simulink model "main"  (Simulink 7.3)
settings: Solver=ode45  StartTime=0.0  StopTime=10.0  RelTol=1e-7
libraries: simulink x2
settings Model: Creator=Sain  LastModifiedBy=Sain

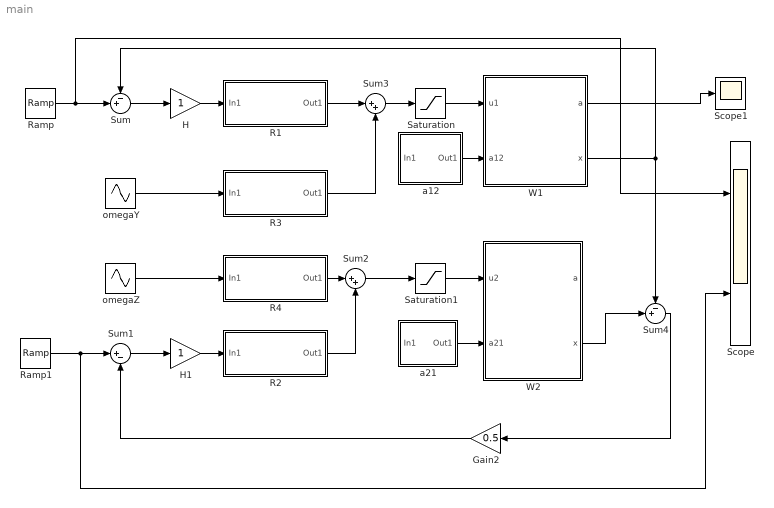
== system main ==
  Gain2 : Gain  Gain=0.5  ParameterDataType=fixdt(1, 16)  ParameterScaling=2^0  OutDataType=fixdt(1, 16)  OutScaling=2^0
  H : Gain  ParameterDataType=fixdt(1, 16)  ParameterScaling=2^0  OutDataType=fixdt(1, 16)  OutScaling=2^0
  H1 : Gain  ParameterDataType=fixdt(1, 16)  ParameterScaling=2^0  OutDataType=fixdt(1, 16)  OutScaling=2^0
  R1 : Subsystem
  R2 : Subsystem
  R3 : Subsystem
  R4 : Subsystem
  Ramp : simulink/Sources/Ramp  SystemSampleTime=-1  slope=60  start=1  X0=0
  Ramp1 : simulink/Sources/Ramp  SystemSampleTime=-1  slope=30  start=2  X0=0
  Saturation : Saturate  UpperLimit=27  LowerLimit=-27  OutDataType=fixdt(1, 16)  OutScaling=2^0
  Saturation1 : Saturate  UpperLimit=27  LowerLimit=-27  OutDataType=fixdt(1, 16)  OutScaling=2^0
  Scope : Scope  NumInputPorts=2
      settings: YMin=-5~-5  YMax=5~5
  Scope1 : Scope
  Sum : Sum  Inputs=-+|  OutDataType=fixdt(1, 16)  OutScaling=2^0
  Sum1 : Sum  Inputs=|+-  OutDataType=fixdt(1, 16)  OutScaling=2^0
  Sum2 : Sum  Inputs=|++  OutDataType=fixdt(1, 16)  OutScaling=2^0
  Sum3 : Sum  Inputs=|++  OutDataType=fixdt(1, 16)  OutScaling=2^0
  Sum4 : Sum  Inputs=-+|  OutDataType=fixdt(1, 16)  OutScaling=2^0
  W1 : Subsystem
  W2 : Subsystem
  a12 : Subsystem
  a21 : Subsystem
  omegaY : Sin  Amplitude=1  Bias=0  Frequency=2  Phase=0  Samples=10  SampleTime=0  Offset=0
  omegaZ : Sin  Amplitude=1  Bias=0  Frequency=2  Phase=0  Samples=10  SampleTime=0  Offset=0
  wires:
  Sum/1 -> H/1
  Sum1/1 -> H1/1
  R2/1(Out1) -> Sum2/2
  R4/1(Out1) -> Sum2/1
  Sum2/1 -> Saturation1/1
  R1/1(Out1) -> Sum3/1
  Sum3/1 -> Saturation/1
  R3/1(Out1) -> Sum3/2
  H/1 -> R1/1(In1)
  Sum4/1 -> Gain2/1
  Gain2/1 -> Sum1/2
  Saturation1/1 -> W2/1(u2)
  a21/1(Out1) -> W2/2(a21)
  Saturation/1 -> W1/1(u1)
  a12/1(Out1) -> W1/2(a12)
  W1/2(x) -> Sum4/1, Sum/1
  W2/2(x) -> Sum4/2
  H1/1 -> R2/1(In1)
  omegaY/1 -> R3/1(In1)
  omegaZ/1 -> R4/1(In1)
  Ramp1/1 -> Scope/2, Sum1/1
  Ramp/1 -> Scope/1, Sum/2
  W1/1(a) -> Scope1/1

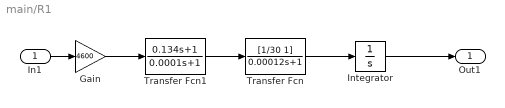
== system main/R1 ==
  In1 : Inport  OutDataType=fixdt(1, 16)  OutScaling=2^0
  Gain : Gain  Gain=4600  ParameterDataType=fixdt(1, 16)  ParameterScaling=2^0  OutDataType=fixdt(1, 16)  OutScaling=2^0
  Integrator : Integrator
  Transfer Fcn : TransferFcn  Numerator=[1/30 1]  Denominator=[0.00012 1]
  Transfer Fcn1 : TransferFcn  Numerator=[0.134 1]  Denominator=[0.0001 1]
  Out1 : Outport  OutDataType=fixdt(1, 16)  OutScaling=2^0
  wires:
  In1/1 -> Gain/1
  Transfer Fcn1/1 -> Transfer Fcn/1
  Transfer Fcn/1 -> Integrator/1
  Integrator/1 -> Out1/1
  Gain/1 -> Transfer Fcn1/1

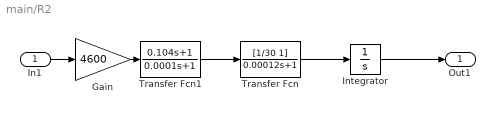
== system main/R2 ==
  In1 : Inport  OutDataType=fixdt(1, 16)  OutScaling=2^0
  Gain : Gain  Gain=4600  ParameterDataType=fixdt(1, 16)  ParameterScaling=2^0  OutDataType=fixdt(1, 16)  OutScaling=2^0
  Integrator : Integrator
  Transfer Fcn : TransferFcn  Numerator=[1/30 1]  Denominator=[0.00012 1]
  Transfer Fcn1 : TransferFcn  Numerator=[0.104 1]  Denominator=[0.0001 1]
  Out1 : Outport  OutDataType=fixdt(1, 16)  OutScaling=2^0
  wires:
  In1/1 -> Gain/1
  Transfer Fcn1/1 -> Transfer Fcn/1
  Transfer Fcn/1 -> Integrator/1
  Integrator/1 -> Out1/1
  Gain/1 -> Transfer Fcn1/1

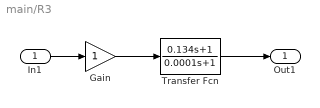
== system main/R3 ==
  In1 : Inport  OutDataType=fixdt(1, 16)  OutScaling=2^0
  Gain : Gain  ParameterDataType=fixdt(1, 16)  ParameterScaling=2^0  OutDataType=fixdt(1, 16)  OutScaling=2^0
  Transfer Fcn : TransferFcn  Numerator=[0.134 1]  Denominator=[0.0001 1]
  Out1 : Outport  OutDataType=fixdt(1, 16)  OutScaling=2^0
  wires:
  In1/1 -> Gain/1
  Gain/1 -> Transfer Fcn/1
  Transfer Fcn/1 -> Out1/1

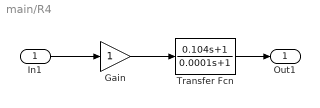
== system main/R4 ==
  In1 : Inport  OutDataType=fixdt(1, 16)  OutScaling=2^0
  Gain : Gain  ParameterDataType=fixdt(1, 16)  ParameterScaling=2^0  OutDataType=fixdt(1, 16)  OutScaling=2^0
  Transfer Fcn : TransferFcn  Numerator=[0.104 1]  Denominator=[0.0001 1]
  Out1 : Outport  OutDataType=fixdt(1, 16)  OutScaling=2^0
  wires:
  Gain/1 -> Transfer Fcn/1
  In1/1 -> Gain/1
  Transfer Fcn/1 -> Out1/1

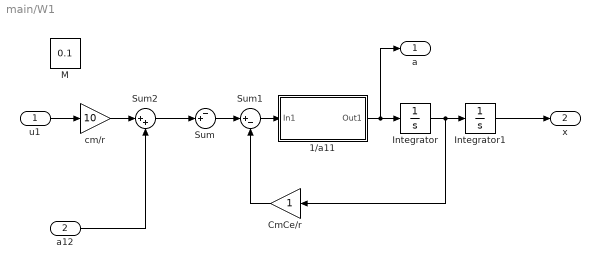
== system main/W1 ==
  u1 : Inport  OutDataType=fixdt(1, 16)  OutScaling=2^0
  a12 : Inport  Port=2  OutDataType=fixdt(1, 16)  OutScaling=2^0
  1/a11 : Subsystem
  CmCe/r : Gain  ParameterDataType=fixdt(1, 16)  ParameterScaling=2^0  OutDataType=fixdt(1, 16)  OutScaling=2^0
  Integrator : Integrator
  Integrator1 : Integrator
  M : Constant  Value=0.1  OutDataType=fixdt(1, 16)  OutScaling=2^0
  Sum : Sum  Inputs=-+|  OutDataType=fixdt(1, 16)  OutScaling=2^0
  Sum1 : Sum  Inputs=|+-  OutDataType=fixdt(1, 16)  OutScaling=2^0
  Sum2 : Sum  Inputs=|++  OutDataType=fixdt(1, 16)  OutScaling=2^0
  cm/r : Gain  Gain=10  ParameterDataType=fixdt(1, 16)  ParameterScaling=2^0  OutDataType=fixdt(1, 16)  OutScaling=2^0
  a : Outport  OutDataType=fixdt(1, 16)  OutScaling=2^0
  x : Outport  Port=2  OutDataType=fixdt(1, 16)  OutScaling=2^0
  wires:
  u1/1 -> cm/r/1
  Integrator/1 -> Integrator1/1, CmCe/r/1
  Integrator1/1 -> x/1
  cm/r/1 -> Sum2/1
  a12/1 -> Sum2/2
  Sum1/1 -> 1/a11/1(In1)
  1/a11/1(Out1) -> Integrator/1, a/1
  Sum2/1 -> Sum/2
  Sum/1 -> Sum1/1
  CmCe/r/1 -> Sum1/2

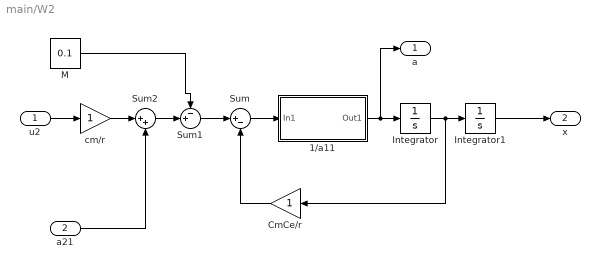
== system main/W2 ==
  u2 : Inport  OutDataType=fixdt(1, 16)  OutScaling=2^0
  a21 : Inport  Port=2  OutDataType=fixdt(1, 16)  OutScaling=2^0
  1/a11 : Subsystem
  CmCe/r : Gain  ParameterDataType=fixdt(1, 16)  ParameterScaling=2^0  OutDataType=fixdt(1, 16)  OutScaling=2^0
  Integrator : Integrator
  Integrator1 : Integrator
  M : Constant  Value=0.1  OutDataType=fixdt(1, 16)  OutScaling=2^0
  Sum : Sum  Inputs=|+-  OutDataType=fixdt(1, 16)  OutScaling=2^0
  Sum1 : Sum  Inputs=-+|  OutDataType=fixdt(1, 16)  OutScaling=2^0
  Sum2 : Sum  Inputs=|++  OutDataType=fixdt(1, 16)  OutScaling=2^0
  cm/r : Gain  ParameterDataType=fixdt(1, 16)  ParameterScaling=2^0  OutDataType=fixdt(1, 16)  OutScaling=2^0
  a : Outport  OutDataType=fixdt(1, 16)  OutScaling=2^0
  x : Outport  Port=2  OutDataType=fixdt(1, 16)  OutScaling=2^0
  wires:
  M/1 -> Sum1/1
  u2/1 -> cm/r/1
  Integrator/1 -> Integrator1/1, CmCe/r/1
  Integrator1/1 -> x/1
  cm/r/1 -> Sum2/1
  a21/1 -> Sum2/2
  Sum/1 -> 1/a11/1(In1)
  CmCe/r/1 -> Sum/2
  1/a11/1(Out1) -> Integrator/1, a/1
  Sum2/1 -> Sum1/2
  Sum1/1 -> Sum/1

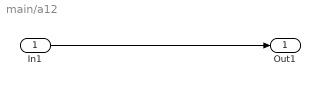
== system main/a12 ==
  In1 : Inport  OutDataType=fixdt(1, 16)  OutScaling=2^0
  Out1 : Outport  OutDataType=fixdt(1, 16)  OutScaling=2^0
  wires:
  In1/1 -> Out1/1

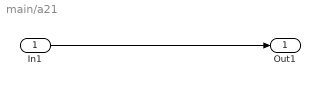
== system main/a21 ==
  In1 : Inport  OutDataType=fixdt(1, 16)  OutScaling=2^0
  Out1 : Outport  OutDataType=fixdt(1, 16)  OutScaling=2^0
  wires:
  In1/1 -> Out1/1

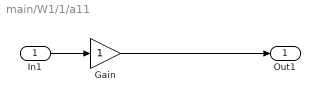
== system main/W1/1/a11 ==
  In1 : Inport  OutDataType=fixdt(1, 16)  OutScaling=2^0
  Gain : Gain  ParameterDataType=fixdt(1, 16)  ParameterScaling=2^0  OutDataType=fixdt(1, 16)  OutScaling=2^0
  Out1 : Outport  OutDataType=fixdt(1, 16)  OutScaling=2^0
  wires:
  In1/1 -> Gain/1
  Gain/1 -> Out1/1

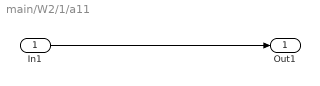
== system main/W2/1/a11 ==
  In1 : Inport  OutDataType=fixdt(1, 16)  OutScaling=2^0
  Out1 : Outport  OutDataType=fixdt(1, 16)  OutScaling=2^0
  wires:
  In1/1 -> Out1/1
